simulink library "BWB_library"  (R2017b)
settings: Solver=VariableStepAuto  StartTime=0.0  StopTime=10.0  RelTol=1e-3
undefined symbols (not defined in the file or in its folder): BWB, BWB_uncoupled, BWBlat, BWBlat1, BWBlon, F, I, Ixx, Iyy, Izz, Light, m, MIL, pqr0, ptp0, Vb0, x0, Xe0
libraries: aerolibasang x4, aerolibwind2 x3, shared6dof x2, aerolibadyn x2, aerolibatmos2 x1
(part 2 of 2)

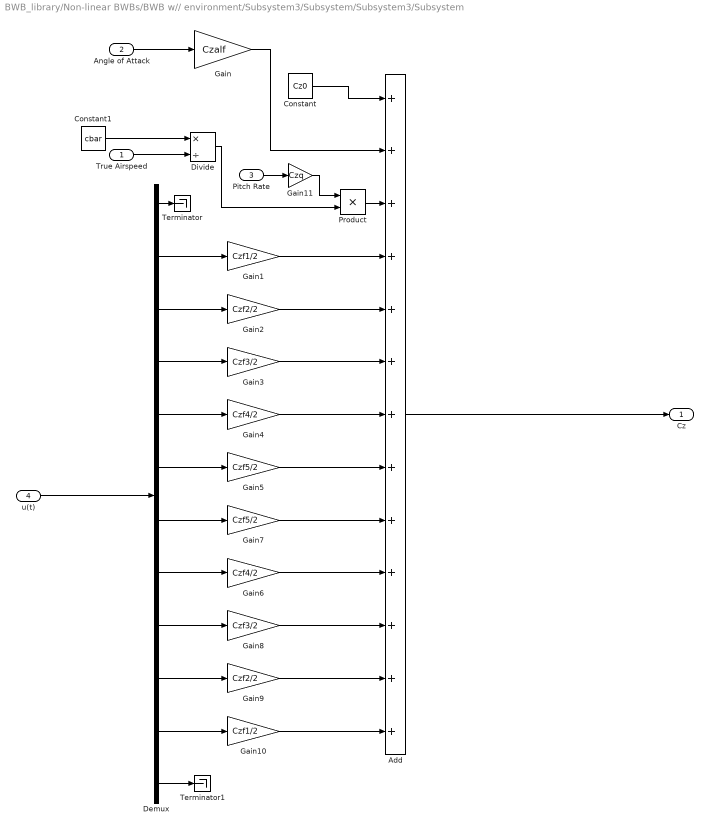
== system BWB_library/Non-linear BWBs/BWB w// environment/Subsystem3/Subsystem/Subsystem3/Subsystem ==
  True Airspeed : Inport
  Angle of Attack : Inport  Port=2
  Pitch Rate : Inport  Port=3
  u(t) : Inport  Port=4
  Add : Sum  Inputs=+++++++++++++
  Constant : Constant  Value=Cz0
  Constant1 : Constant  Value=cbar
  Demux : Demux  Outputs=12
  Divide : Product  Inputs=*/
  Gain : Gain  Gain=Czalf
  Gain1 : Gain  Gain=Czf1/2
  Gain10 : Gain  Gain=Czf1/2
  Gain11 : Gain  Gain=Czq
  Gain2 : Gain  Gain=Czf2/2
  Gain3 : Gain  Gain=Czf3/2
  Gain4 : Gain  Gain=Czf4/2
  Gain5 : Gain  Gain=Czf5/2
  Gain6 : Gain  Gain=Czf4/2
  Gain7 : Gain  Gain=Czf5/2
  Gain8 : Gain  Gain=Czf3/2
  Gain9 : Gain  Gain=Czf2/2
  Product : Product
  Terminator : Terminator
  Terminator1 : Terminator
  Cz : Outport
  wires:
  Add/1 -> Cz/1
  Gain/1 -> Add/2
  True Airspeed/1 -> Divide/2
  Angle of Attack/1 -> Gain/1
  Constant/1 -> Add/1
  Gain9/1 -> Add/12
  Gain7/1 -> Add/9
  Demux/2 -> Gain1/1
  Gain6/1 -> Add/10
  Demux/11 -> Gain10/1
  Demux/6 -> Gain5/1
  Demux/4 -> Gain3/1
  Demux/5 -> Gain4/1
  Divide/1 -> Product/2
  Demux/7 -> Gain7/1
  Gain1/1 -> Add/4
  Gain2/1 -> Add/5
  Gain8/1 -> Add/11
  Gain5/1 -> Add/8
  Demux/8 -> Gain6/1
  Demux/9 -> Gain8/1
  Gain3/1 -> Add/6
  Demux/10 -> Gain9/1
  Demux/3 -> Gain2/1
  Gain10/1 -> Add/13
  Constant1/1 -> Divide/1
  Gain4/1 -> Add/7
  Demux/1 -> Terminator/1
  Demux/12 -> Terminator1/1
  u(t)/1 -> Demux/1
  Gain11/1 -> Product/1
  Pitch Rate/1 -> Gain11/1
  Product/1 -> Add/3

== system BWB_library/Non-linear BWBs/BWB w// environment/Subsystem3/Subsystem/Subsystem3/Subsystem1 ==
  Cz : Inport
  Add : Sum  Inputs=+-+
  Constant : Constant  Value=Cx0
  Gain : Gain  Gain=Cx1
  Gain1 : Gain  Gain=Cx2
  Gain2 : Gain  Gain=-1
  Math Function : Math  Operator=square  SaturateOnIntegerOverflow=on
  Cx : Outport
  wires:
  Math Function/1 -> Gain1/1
  Gain1/1 -> Add/3
  Gain/1 -> Add/2
  Gain2/1 -> Cx/1
  Constant/1 -> Add/1
  Add/1 -> Gain2/1
  Cz/1 -> Math Function/1, Gain/1

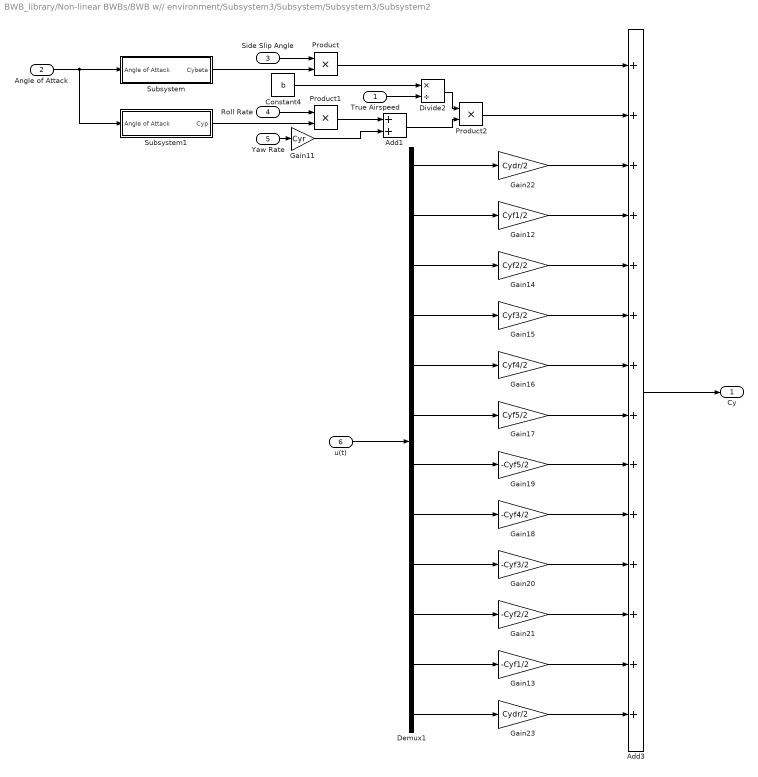
== system BWB_library/Non-linear BWBs/BWB w// environment/Subsystem3/Subsystem/Subsystem3/Subsystem2 ==
  True Airspeed : Inport
  Angle of Attack : Inport  Port=2
  Side Slip Angle : Inport  Port=3
  Roll Rate : Inport  Port=4
  Yaw Rate : Inport  Port=5
  u(t) : Inport  Port=6
  Add1 : Sum
  Add3 : Sum  Inputs=++++++++++++++
  Constant4 : Constant  Value=b
  Demux1 : Demux  Outputs=12
  Divide2 : Product  Inputs=*/
  Gain11 : Gain  Gain=Cyr
  Gain12 : Gain  Gain=Cyf1/2
  Gain13 : Gain  Gain=-Cyf1/2
  Gain14 : Gain  Gain=Cyf2/2
  Gain15 : Gain  Gain=Cyf3/2
  Gain16 : Gain  Gain=Cyf4/2
  Gain17 : Gain  Gain=Cyf5/2
  Gain18 : Gain  Gain=-Cyf4/2
  Gain19 : Gain  Gain=-Cyf5/2
  Gain20 : Gain  Gain=-Cyf3/2
  Gain21 : Gain  Gain=-Cyf2/2
  Gain22 : Gain  Gain=Cydr/2
  Gain23 : Gain  Gain=Cydr/2
  Product : Product
  Product1 : Product
  Product2 : Product
  Subsystem : Subsystem
  Subsystem1 : Subsystem
  Cy : Outport
  wires:
  Side Slip Angle/1 -> Product/1
  Product/1 -> Add3/1
  Angle of Attack/1 -> Subsystem1/1(Angle of Attack), Subsystem/1(Angle of Attack)
  Subsystem/1(Cybeta) -> Product/2
  Subsystem1/1(Cyp) -> Product1/2
  Roll Rate/1 -> Product1/1
  Product1/1 -> Add1/1
  Gain11/1 -> Add1/2
  Yaw Rate/1 -> Gain11/1
  Add1/1 -> Product2/2
  Divide2/1 -> Product2/1
  True Airspeed/1 -> Divide2/2
  Constant4/1 -> Divide2/1
  Product2/1 -> Add3/2
  Demux1/6 -> Gain17/1
  Gain18/1 -> Add3/10
  Demux1/2 -> Gain12/1
  Gain19/1 -> Add3/9
  Demux1/4 -> Gain15/1
  Demux1/7 -> Gain19/1
  Demux1/5 -> Gain16/1
  Demux1/9 -> Gain20/1
  u(t)/1 -> Demux1/1
  Gain15/1 -> Add3/6
  Gain21/1 -> Add3/12
  Demux1/8 -> Gain18/1
  Gain17/1 -> Add3/8
  Gain20/1 -> Add3/11
  Demux1/11 -> Gain13/1
  Gain12/1 -> Add3/4
  Demux1/3 -> Gain14/1
  Demux1/1 -> Gain22/1
  Gain13/1 -> Add3/13
  Gain16/1 -> Add3/7
  Gain14/1 -> Add3/5
  Demux1/10 -> Gain21/1
  Demux1/12 -> Gain23/1
  Gain22/1 -> Add3/3
  Gain23/1 -> Add3/14
  Add3/1 -> Cy/1

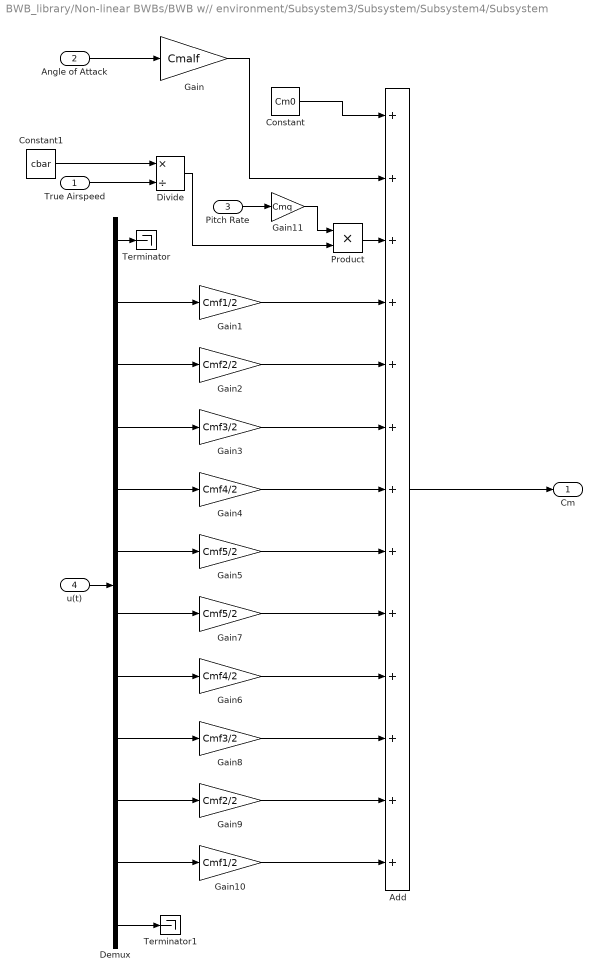
== system BWB_library/Non-linear BWBs/BWB w// environment/Subsystem3/Subsystem/Subsystem4/Subsystem ==
  True Airspeed : Inport
  Angle of Attack : Inport  Port=2
  Pitch Rate : Inport  Port=3
  u(t) : Inport  Port=4
  Add : Sum  Inputs=+++++++++++++
  Constant : Constant  Value=Cm0
  Constant1 : Constant  Value=cbar
  Demux : Demux  Outputs=12
  Divide : Product  Inputs=*/
  Gain : Gain  Gain=Cmalf
  Gain1 : Gain  Gain=Cmf1/2
  Gain10 : Gain  Gain=Cmf1/2
  Gain11 : Gain  Gain=Cmq
  Gain2 : Gain  Gain=Cmf2/2
  Gain3 : Gain  Gain=Cmf3/2
  Gain4 : Gain  Gain=Cmf4/2
  Gain5 : Gain  Gain=Cmf5/2
  Gain6 : Gain  Gain=Cmf4/2
  Gain7 : Gain  Gain=Cmf5/2
  Gain8 : Gain  Gain=Cmf3/2
  Gain9 : Gain  Gain=Cmf2/2
  Product : Product
  Terminator : Terminator
  Terminator1 : Terminator
  Cm : Outport
  wires:
  Add/1 -> Cm/1
  Gain/1 -> Add/2
  True Airspeed/1 -> Divide/2
  Angle of Attack/1 -> Gain/1
  Constant/1 -> Add/1
  Gain9/1 -> Add/12
  Gain7/1 -> Add/9
  Demux/2 -> Gain1/1
  Gain6/1 -> Add/10
  Demux/11 -> Gain10/1
  Demux/6 -> Gain5/1
  Demux/4 -> Gain3/1
  Demux/5 -> Gain4/1
  Divide/1 -> Product/2
  Demux/7 -> Gain7/1
  Gain1/1 -> Add/4
  Gain2/1 -> Add/5
  Gain8/1 -> Add/11
  Gain5/1 -> Add/8
  Demux/8 -> Gain6/1
  Demux/9 -> Gain8/1
  Gain3/1 -> Add/6
  Demux/10 -> Gain9/1
  Demux/3 -> Gain2/1
  Gain10/1 -> Add/13
  Constant1/1 -> Divide/1
  Gain4/1 -> Add/7
  Demux/1 -> Terminator/1
  Demux/12 -> Terminator1/1
  u(t)/1 -> Demux/1
  Gain11/1 -> Product/1
  Pitch Rate/1 -> Gain11/1
  Product/1 -> Add/3

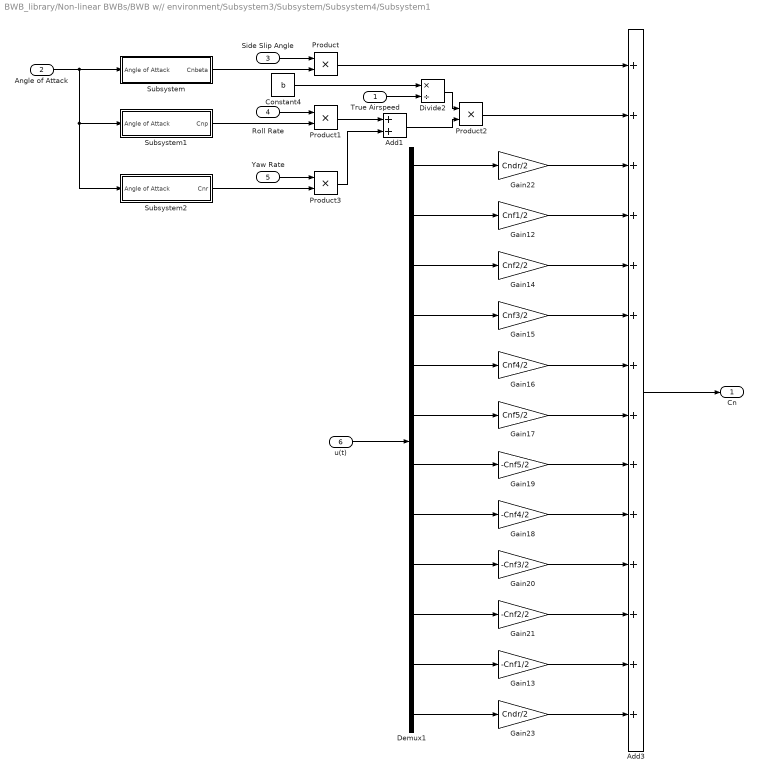
== system BWB_library/Non-linear BWBs/BWB w// environment/Subsystem3/Subsystem/Subsystem4/Subsystem1 ==
  True Airspeed : Inport
  Angle of Attack : Inport  Port=2
  Side Slip Angle : Inport  Port=3
  Roll Rate : Inport  Port=4
  Yaw Rate : Inport  Port=5
  u(t) : Inport  Port=6
  Add1 : Sum
  Add3 : Sum  Inputs=++++++++++++++
  Constant4 : Constant  Value=b
  Demux1 : Demux  Outputs=12
  Divide2 : Product  Inputs=*/
  Gain12 : Gain  Gain=Cnf1/2
  Gain13 : Gain  Gain=-Cnf1/2
  Gain14 : Gain  Gain=Cnf2/2
  Gain15 : Gain  Gain=Cnf3/2
  Gain16 : Gain  Gain=Cnf4/2
  Gain17 : Gain  Gain=Cnf5/2
  Gain18 : Gain  Gain=-Cnf4/2
  Gain19 : Gain  Gain=-Cnf5/2
  Gain20 : Gain  Gain=-Cnf3/2
  Gain21 : Gain  Gain=-Cnf2/2
  Gain22 : Gain  Gain=Cndr/2
  Gain23 : Gain  Gain=Cndr/2
  Product{,1..3} (4 alike) : Product
  Subsystem : Subsystem
  Subsystem1 : Subsystem
  Subsystem2 : Subsystem
  Cn : Outport
  wires:
  Side Slip Angle/1 -> Product/1
  Product/1 -> Add3/1
  Angle of Attack/1 -> Subsystem1/1(Angle of Attack), Subsystem2/1(Angle of Attack), Subsystem/1(Angle of Attack)
  Subsystem/1(Cnbeta) -> Product/2
  Subsystem1/1(Cnp) -> Product1/2
  Roll Rate/1 -> Product1/1
  Product1/1 -> Add1/1
  Product3/1 -> Add1/2
  Yaw Rate/1 -> Product3/1
  Add1/1 -> Product2/2
  Divide2/1 -> Product2/1
  True Airspeed/1 -> Divide2/2
  Constant4/1 -> Divide2/1
  Product2/1 -> Add3/2
  Demux1/6 -> Gain17/1
  Gain18/1 -> Add3/10
  Demux1/2 -> Gain12/1
  Gain19/1 -> Add3/9
  Demux1/4 -> Gain15/1
  Demux1/7 -> Gain19/1
  Demux1/5 -> Gain16/1
  Demux1/9 -> Gain20/1
  u(t)/1 -> Demux1/1
  Gain15/1 -> Add3/6
  Gain21/1 -> Add3/12
  Demux1/8 -> Gain18/1
  Gain17/1 -> Add3/8
  Gain20/1 -> Add3/11
  Demux1/11 -> Gain13/1
  Gain12/1 -> Add3/4
  Demux1/3 -> Gain14/1
  Demux1/1 -> Gain22/1
  Gain13/1 -> Add3/13
  Gain16/1 -> Add3/7
  Gain14/1 -> Add3/5
  Demux1/10 -> Gain21/1
  Demux1/12 -> Gain23/1
  Gain22/1 -> Add3/3
  Gain23/1 -> Add3/14
  Add3/1 -> Cn/1
  Subsystem2/1(Cnr) -> Product3/2

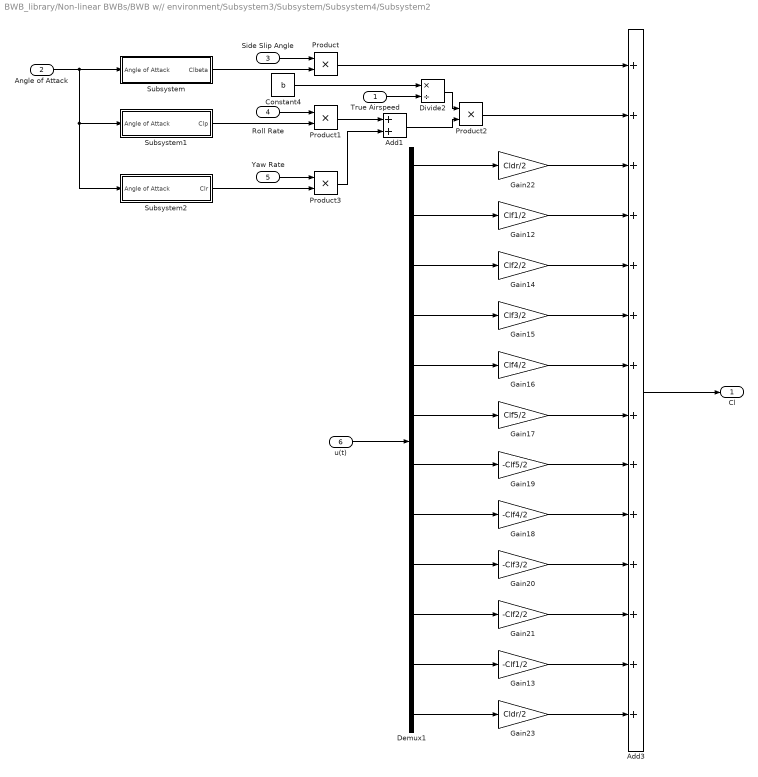
== system BWB_library/Non-linear BWBs/BWB w// environment/Subsystem3/Subsystem/Subsystem4/Subsystem2 ==
  True Airspeed : Inport
  Angle of Attack : Inport  Port=2
  Side Slip Angle : Inport  Port=3
  Roll Rate : Inport  Port=4
  Yaw Rate : Inport  Port=5
  u(t) : Inport  Port=6
  Add1 : Sum
  Add3 : Sum  Inputs=++++++++++++++
  Constant4 : Constant  Value=b
  Demux1 : Demux  Outputs=12
  Divide2 : Product  Inputs=*/
  Gain12 : Gain  Gain=Clf1/2
  Gain13 : Gain  Gain=-Clf1/2
  Gain14 : Gain  Gain=Clf2/2
  Gain15 : Gain  Gain=Clf3/2
  Gain16 : Gain  Gain=Clf4/2
  Gain17 : Gain  Gain=Clf5/2
  Gain18 : Gain  Gain=-Clf4/2
  Gain19 : Gain  Gain=-Clf5/2
  Gain20 : Gain  Gain=-Clf3/2
  Gain21 : Gain  Gain=-Clf2/2
  Gain22 : Gain  Gain=Cldr/2
  Gain23 : Gain  Gain=Cldr/2
  Product{,1..3} (4 alike) : Product
  Subsystem : Subsystem
  Subsystem1 : Subsystem
  Subsystem2 : Subsystem
  Cl : Outport
  wires:
  Side Slip Angle/1 -> Product/1
  Product/1 -> Add3/1
  Angle of Attack/1 -> Subsystem1/1(Angle of Attack), Subsystem2/1(Angle of Attack), Subsystem/1(Angle of Attack)
  Subsystem/1(Clbeta) -> Product/2
  Subsystem1/1(Clp) -> Product1/2
  Roll Rate/1 -> Product1/1
  Product1/1 -> Add1/1
  Product3/1 -> Add1/2
  Yaw Rate/1 -> Product3/1
  Add1/1 -> Product2/2
  Divide2/1 -> Product2/1
  True Airspeed/1 -> Divide2/2
  Constant4/1 -> Divide2/1
  Product2/1 -> Add3/2
  Demux1/6 -> Gain17/1
  Gain18/1 -> Add3/10
  Demux1/2 -> Gain12/1
  Gain19/1 -> Add3/9
  Demux1/4 -> Gain15/1
  Demux1/7 -> Gain19/1
  Demux1/5 -> Gain16/1
  Demux1/9 -> Gain20/1
  u(t)/1 -> Demux1/1
  Gain15/1 -> Add3/6
  Gain21/1 -> Add3/12
  Demux1/8 -> Gain18/1
  Gain17/1 -> Add3/8
  Gain20/1 -> Add3/11
  Demux1/11 -> Gain13/1
  Gain12/1 -> Add3/4
  Demux1/3 -> Gain14/1
  Demux1/1 -> Gain22/1
  Gain13/1 -> Add3/13
  Gain16/1 -> Add3/7
  Gain14/1 -> Add3/5
  Demux1/10 -> Gain21/1
  Demux1/12 -> Gain23/1
  Gain22/1 -> Add3/3
  Gain23/1 -> Add3/14
  Add3/1 -> Cl/1
  Subsystem2/1(Clr) -> Product3/2

== system BWB_library/Non-linear BWBs/BWB non-linear/Subsystem3/Subsystem/Subsystem3/Subsystem2/Subsystem ==
  Angle of Attack : Inport
  Add1 : Sum
  Constant2 : Constant  Value=Cybet0
  Gain11 : Gain  Gain=Cybetalf
  Cybeta : Outport
  wires:
  Constant2/1 -> Add1/1
  Add1/1 -> Cybeta/1
  Angle of Attack/1 -> Gain11/1
  Gain11/1 -> Add1/2

== system BWB_library/Non-linear BWBs/BWB non-linear/Subsystem3/Subsystem/Subsystem3/Subsystem2/Subsystem1 ==
  Angle of Attack : Inport
  Add1 : Sum
  Constant2 : Constant  Value=Cyp0
  Gain11 : Gain  Gain=Cypalf
  Cyp : Outport
  wires:
  Constant2/1 -> Add1/1
  Add1/1 -> Cyp/1
  Angle of Attack/1 -> Gain11/1
  Gain11/1 -> Add1/2

== system BWB_library/Non-linear BWBs/BWB non-linear/Subsystem3/Subsystem/Subsystem4/Subsystem1/Subsystem ==
  Angle of Attack : Inport
  Add1 : Sum
  Constant2 : Constant  Value=Cnbet0
  Gain11 : Gain  Gain=Cnbetalf
  Cnbeta : Outport
  wires:
  Constant2/1 -> Add1/1
  Add1/1 -> Cnbeta/1
  Angle of Attack/1 -> Gain11/1
  Gain11/1 -> Add1/2

== system BWB_library/Non-linear BWBs/BWB non-linear/Subsystem3/Subsystem/Subsystem4/Subsystem1/Subsystem1 ==
  Angle of Attack : Inport
  Add1 : Sum
  Constant2 : Constant  Value=Cnp0
  Gain11 : Gain  Gain=Cnpalf
  Cnp : Outport
  wires:
  Constant2/1 -> Add1/1
  Add1/1 -> Cnp/1
  Angle of Attack/1 -> Gain11/1
  Gain11/1 -> Add1/2

== system BWB_library/Non-linear BWBs/BWB non-linear/Subsystem3/Subsystem/Subsystem4/Subsystem1/Subsystem2 ==
  Angle of Attack : Inport
  Add1 : Sum
  Constant2 : Constant  Value=Cnr0
  Gain11 : Gain  Gain=Cnralf
  Cnr : Outport
  wires:
  Constant2/1 -> Add1/1
  Add1/1 -> Cnr/1
  Angle of Attack/1 -> Gain11/1
  Gain11/1 -> Add1/2

== system BWB_library/Non-linear BWBs/BWB non-linear/Subsystem3/Subsystem/Subsystem4/Subsystem2/Subsystem ==
  Angle of Attack : Inport
  Add1 : Sum
  Constant2 : Constant  Value=Clbet0
  Gain11 : Gain  Gain=Clbetalf
  Clbeta : Outport
  wires:
  Constant2/1 -> Add1/1
  Add1/1 -> Clbeta/1
  Angle of Attack/1 -> Gain11/1
  Gain11/1 -> Add1/2

== system BWB_library/Non-linear BWBs/BWB non-linear/Subsystem3/Subsystem/Subsystem4/Subsystem2/Subsystem1 ==
  Angle of Attack : Inport
  Add1 : Sum
  Constant2 : Constant  Value=Clp0
  Gain11 : Gain  Gain=Clpalf
  Clp : Outport
  wires:
  Constant2/1 -> Add1/1
  Add1/1 -> Clp/1
  Angle of Attack/1 -> Gain11/1
  Gain11/1 -> Add1/2

== system BWB_library/Non-linear BWBs/BWB non-linear/Subsystem3/Subsystem/Subsystem4/Subsystem2/Subsystem2 ==
  Angle of Attack : Inport
  Add1 : Sum
  Constant2 : Constant  Value=Clr0
  Gain11 : Gain  Gain=Clralf
  Clr : Outport
  wires:
  Constant2/1 -> Add1/1
  Add1/1 -> Clr/1
  Angle of Attack/1 -> Gain11/1
  Gain11/1 -> Add1/2

== system BWB_library/Non-linear BWBs/BWB w// environment/Subsystem3/Subsystem/Subsystem3/Subsystem2/Subsystem ==
  Angle of Attack : Inport
  Add1 : Sum
  Constant2 : Constant  Value=Cybet0
  Gain11 : Gain  Gain=Cybetalf
  Cybeta : Outport
  wires:
  Constant2/1 -> Add1/1
  Add1/1 -> Cybeta/1
  Angle of Attack/1 -> Gain11/1
  Gain11/1 -> Add1/2

== system BWB_library/Non-linear BWBs/BWB w// environment/Subsystem3/Subsystem/Subsystem3/Subsystem2/Subsystem1 ==
  Angle of Attack : Inport
  Add1 : Sum
  Constant2 : Constant  Value=Cyp0
  Gain11 : Gain  Gain=Cypalf
  Cyp : Outport
  wires:
  Constant2/1 -> Add1/1
  Add1/1 -> Cyp/1
  Angle of Attack/1 -> Gain11/1
  Gain11/1 -> Add1/2

== system BWB_library/Non-linear BWBs/BWB w// environment/Subsystem3/Subsystem/Subsystem4/Subsystem1/Subsystem ==
  Angle of Attack : Inport
  Add1 : Sum
  Constant2 : Constant  Value=Cnbet0
  Gain11 : Gain  Gain=Cnbetalf
  Cnbeta : Outport
  wires:
  Constant2/1 -> Add1/1
  Add1/1 -> Cnbeta/1
  Angle of Attack/1 -> Gain11/1
  Gain11/1 -> Add1/2

== system BWB_library/Non-linear BWBs/BWB w// environment/Subsystem3/Subsystem/Subsystem4/Subsystem1/Subsystem1 ==
  Angle of Attack : Inport
  Add1 : Sum
  Constant2 : Constant  Value=Cnp0
  Gain11 : Gain  Gain=Cnpalf
  Cnp : Outport
  wires:
  Constant2/1 -> Add1/1
  Add1/1 -> Cnp/1
  Angle of Attack/1 -> Gain11/1
  Gain11/1 -> Add1/2

== system BWB_library/Non-linear BWBs/BWB w// environment/Subsystem3/Subsystem/Subsystem4/Subsystem1/Subsystem2 ==
  Angle of Attack : Inport
  Add1 : Sum
  Constant2 : Constant  Value=Cnr0
  Gain11 : Gain  Gain=Cnralf
  Cnr : Outport
  wires:
  Constant2/1 -> Add1/1
  Add1/1 -> Cnr/1
  Angle of Attack/1 -> Gain11/1
  Gain11/1 -> Add1/2

== system BWB_library/Non-linear BWBs/BWB w// environment/Subsystem3/Subsystem/Subsystem4/Subsystem2/Subsystem ==
  Angle of Attack : Inport
  Add1 : Sum
  Constant2 : Constant  Value=Clbet0
  Gain11 : Gain  Gain=Clbetalf
  Clbeta : Outport
  wires:
  Constant2/1 -> Add1/1
  Add1/1 -> Clbeta/1
  Angle of Attack/1 -> Gain11/1
  Gain11/1 -> Add1/2

== system BWB_library/Non-linear BWBs/BWB w// environment/Subsystem3/Subsystem/Subsystem4/Subsystem2/Subsystem1 ==
  Angle of Attack : Inport
  Add1 : Sum
  Constant2 : Constant  Value=Clp0
  Gain11 : Gain  Gain=Clpalf
  Clp : Outport
  wires:
  Constant2/1 -> Add1/1
  Add1/1 -> Clp/1
  Angle of Attack/1 -> Gain11/1
  Gain11/1 -> Add1/2

== system BWB_library/Non-linear BWBs/BWB w// environment/Subsystem3/Subsystem/Subsystem4/Subsystem2/Subsystem2 ==
  Angle of Attack : Inport
  Add1 : Sum
  Constant2 : Constant  Value=Clr0
  Gain11 : Gain  Gain=Clralf
  Clr : Outport
  wires:
  Constant2/1 -> Add1/1
  Add1/1 -> Clr/1
  Angle of Attack/1 -> Gain11/1
  Gain11/1 -> Add1/2
